simulink model "Model2"  (R2018b)
settings: Solver=VariableStepAuto  StartTime=0.0  StopTime=10.0  RelTol=1e-3
values from neighbouring files (symbols this model uses):
  P = 0    [Model.m]
settings Model: Creator=Fabi Kadir  LastModifiedBy=Fabi Kadir

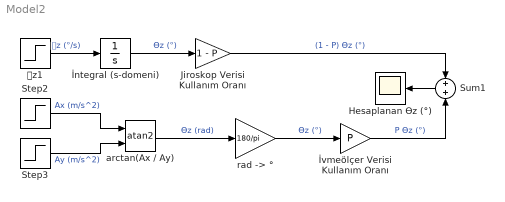
== system Model2 ==
  Hesaplanan Өz (°) : Scope
  Jiroskop Verisi Kullanım Oranı : Gain  Gain=1 - P
  Step2 : Step  SampleTime=0
  Step3 : Step  SampleTime=0
  Sum1 : Sum  Inputs=+|+
  arctan(Ax / Ay) : Trigonometry  Operator=atan2
  "rad -> °" : Gain  Gain=180/pi
  İntegral (s-domeni) : Integrator
  İvmeölçer Verisi Kullanım Oranı : Gain  Gain=P
  Ꞷz1 : Step  SampleTime=0
  wires:
  Step2/1 -> arctan(Ax / Ay)/1  "Ax (m/s^2)"
  arctan(Ax / Ay)/1 -> "rad -> °"/1  "Өz (rad)"
  Step3/1 -> arctan(Ax / Ay)/2  "Ay (m/s^2)"
  Sum1/1 -> Hesaplanan Өz (°)/1
  Jiroskop Verisi Kullanım Oranı/1 -> Sum1/1  "(1 - P) Өz (°)"
  "rad -> °"/1 -> İvmeölçer Verisi Kullanım Oranı/1  "Өz (°)"
  İntegral (s-domeni)/1 -> Jiroskop Verisi Kullanım Oranı/1  "Өz (°)"
  İvmeölçer Verisi Kullanım Oranı/1 -> Sum1/2  "P Өz (°)"
  Ꞷz1/1 -> İntegral (s-domeni)/1  "Ꞷz (°/s)"
